simulink model "P702_NI_SoftECU"  (R2019a)
settings: Solver=ode1  StartTime=0.0  StopTime=Inf  FixedStep=0.001  RelTol=1e-3  EnableMultiTasking=on
PreLoadFcn:
  | run '.\VeriStand_BlockSet\NIVeriStandAddPaths.m'
undefined symbols (not defined in the file or in its folder): magnitude
libraries: simulink x83, simulink_extras x1
(part 10 of 76)

== system P702_NI_SoftECU/Input/BCM/Body_Info_4_0x242 ==
  BattULo_I_Actl : S-Function  Priority=1  FunctionName=NIVeriStandIO  Parameters=width dtype portnum stime stype btype  SFunctionDeploymentMode=off  EnableBusSupport=off  mask(NI VeriStand Inport){portnum=1, width=-1, stime=-1, dtype=auto, stype=auto, btype=1}
      mask prompts: portnum "Port number:"; width "Port dimensions (-1 for dynamically sized):"; stime "Sample time (-1 for inherited):"; dtype "Data type:"; stype "Signal type:"; btype "Block type:"
      mask help: Use this inport on any level of nested subsystems to allow NI VeriStand software to map signals to it.
      mask init:
      | NIVeriStandIO_init;
      settings: CopyFcn=NIVeriStand_MDL_functions('', 'IO_copy');  DeleteFcn=NIVeriStand_MDL_functions('', 'IO_delete');  MoveFcn=set_param(gcb, 'Mask', 'on');
      mask Callback portnum: NIVeriStand_MDL_functions('', 'IO_setportnum');
      mask TypeOptions dtype: auto | double | single | int8 | uint8 | int16 | uint16 | int32 | uint32 | boolean
      mask Callback dtype: NIVeriStand_MDL_functions('', 'IO_booleansignal');
      mask TypeOptions stype: auto | real | complex
      mask Display:
      | patch([-x x], [-y y], [.90980 .81960 .32156]);
      | plot([xrad -x x xrad], [yrad -y y yrad]);
      | fprintf('NI In%d', portnum);
  BattULo_U_Actl : S-Function  Priority=2  FunctionName=NIVeriStandIO  Parameters=width dtype portnum stime stype btype  SFunctionDeploymentMode=off  EnableBusSupport=off  mask(NI VeriStand Inport){portnum=2, width=-1, stime=-1, dtype=auto, stype=auto, btype=1}
      mask prompts: portnum "Port number:"; width "Port dimensions (-1 for dynamically sized):"; stime "Sample time (-1 for inherited):"; dtype "Data type:"; stype "Signal type:"; btype "Block type:"
      mask help: Use this inport on any level of nested subsystems to allow NI VeriStand software to map signals to it.
      mask init:
      | NIVeriStandIO_init;
      settings: CopyFcn=NIVeriStand_MDL_functions('', 'IO_copy');  DeleteFcn=NIVeriStand_MDL_functions('', 'IO_delete');  MoveFcn=set_param(gcb, 'Mask', 'on');
      mask Callback portnum: NIVeriStand_MDL_functions('', 'IO_setportnum');
      mask TypeOptions dtype: auto | double | single | int8 | uint8 | int16 | uint16 | int32 | uint32 | boolean
      mask Callback dtype: NIVeriStand_MDL_functions('', 'IO_booleansignal');
      mask TypeOptions stype: auto | real | complex
      mask Display:
      | patch([-x x], [-y y], [.90980 .81960 .32156]);
      | plot([xrad -x x xrad], [yrad -y y yrad]);
      | fprintf('NI In%d', portnum);
  BrkTrnShifLck_B_Stat : S-Function  Priority=3  FunctionName=NIVeriStandIO  Parameters=width dtype portnum stime stype btype  SFunctionDeploymentMode=off  EnableBusSupport=off  mask(NI VeriStand Inport){portnum=3, width=-1, stime=-1, dtype=auto, stype=auto, btype=1}
      mask prompts: portnum "Port number:"; width "Port dimensions (-1 for dynamically sized):"; stime "Sample time (-1 for inherited):"; dtype "Data type:"; stype "Signal type:"; btype "Block type:"
      mask help: Use this inport on any level of nested subsystems to allow NI VeriStand software to map signals to it.
      mask init:
      | NIVeriStandIO_init;
      settings: CopyFcn=NIVeriStand_MDL_functions('', 'IO_copy');  DeleteFcn=NIVeriStand_MDL_functions('', 'IO_delete');  MoveFcn=set_param(gcb, 'Mask', 'on');
      mask Callback portnum: NIVeriStand_MDL_functions('', 'IO_setportnum');
      mask TypeOptions dtype: auto | double | single | int8 | uint8 | int16 | uint16 | int32 | uint32 | boolean
      mask Callback dtype: NIVeriStand_MDL_functions('', 'IO_booleansignal');
      mask TypeOptions stype: auto | real | complex
      mask Display:
      | patch([-x x], [-y y], [.90980 .81960 .32156]);
      | plot([xrad -x x xrad], [yrad -y y yrad]);
      | fprintf('NI In%d', portnum);
  Bus_Sig : BusCreator  Inputs=15
  DcacElPw_D_Rq : S-Function  Priority=4  FunctionName=NIVeriStandIO  Parameters=width dtype portnum stime stype btype  SFunctionDeploymentMode=off  EnableBusSupport=off  mask(NI VeriStand Inport){portnum=4, width=-1, stime=-1, dtype=auto, stype=auto, btype=1}
      mask prompts: portnum "Port number:"; width "Port dimensions (-1 for dynamically sized):"; stime "Sample time (-1 for inherited):"; dtype "Data type:"; stype "Signal type:"; btype "Block type:"
      mask help: Use this inport on any level of nested subsystems to allow NI VeriStand software to map signals to it.
      mask init:
      | NIVeriStandIO_init;
      settings: CopyFcn=NIVeriStand_MDL_functions('', 'IO_copy');  DeleteFcn=NIVeriStand_MDL_functions('', 'IO_delete');  MoveFcn=set_param(gcb, 'Mask', 'on');
      mask Callback portnum: NIVeriStand_MDL_functions('', 'IO_setportnum');
      mask TypeOptions dtype: auto | double | single | int8 | uint8 | int16 | uint16 | int32 | uint32 | boolean
      mask Callback dtype: NIVeriStand_MDL_functions('', 'IO_booleansignal');
      mask TypeOptions stype: auto | real | complex
      mask Display:
      | patch([-x x], [-y y], [.90980 .81960 .32156]);
      | plot([xrad -x x xrad], [yrad -y y yrad]);
      | fprintf('NI In%d', portnum);
  DriverCrankingReq : S-Function  Priority=5  FunctionName=NIVeriStandIO  Parameters=width dtype portnum stime stype btype  SFunctionDeploymentMode=off  EnableBusSupport=off  mask(NI VeriStand Inport){portnum=5, width=-1, stime=-1, dtype=auto, stype=auto, btype=1}
      mask prompts: portnum "Port number:"; width "Port dimensions (-1 for dynamically sized):"; stime "Sample time (-1 for inherited):"; dtype "Data type:"; stype "Signal type:"; btype "Block type:"
      mask help: Use this inport on any level of nested subsystems to allow NI VeriStand software to map signals to it.
      mask init:
      | NIVeriStandIO_init;
      settings: CopyFcn=NIVeriStand_MDL_functions('', 'IO_copy');  DeleteFcn=NIVeriStand_MDL_functions('', 'IO_delete');  MoveFcn=set_param(gcb, 'Mask', 'on');
      mask Callback portnum: NIVeriStand_MDL_functions('', 'IO_setportnum');
      mask TypeOptions dtype: auto | double | single | int8 | uint8 | int16 | uint16 | int32 | uint32 | boolean
      mask Callback dtype: NIVeriStand_MDL_functions('', 'IO_booleansignal');
      mask TypeOptions stype: auto | real | complex
      mask Display:
      | patch([-x x], [-y y], [.90980 .81960 .32156]);
      | plot([xrad -x x xrad], [yrad -y y yrad]);
      | fprintf('NI In%d', portnum);
  EngOff_T_Actl : S-Function  Priority=6  FunctionName=NIVeriStandIO  Parameters=width dtype portnum stime stype btype  SFunctionDeploymentMode=off  EnableBusSupport=off  mask(NI VeriStand Inport){portnum=6, width=-1, stime=-1, dtype=auto, stype=auto, btype=1}
      mask prompts: portnum "Port number:"; width "Port dimensions (-1 for dynamically sized):"; stime "Sample time (-1 for inherited):"; dtype "Data type:"; stype "Signal type:"; btype "Block type:"
      mask help: Use this inport on any level of nested subsystems to allow NI VeriStand software to map signals to it.
      mask init:
      | NIVeriStandIO_init;
      settings: CopyFcn=NIVeriStand_MDL_functions('', 'IO_copy');  DeleteFcn=NIVeriStand_MDL_functions('', 'IO_delete');  MoveFcn=set_param(gcb, 'Mask', 'on');
      mask Callback portnum: NIVeriStand_MDL_functions('', 'IO_setportnum');
      mask TypeOptions dtype: auto | double | single | int8 | uint8 | int16 | uint16 | int32 | uint32 | boolean
      mask Callback dtype: NIVeriStand_MDL_functions('', 'IO_booleansignal');
      mask TypeOptions stype: auto | real | complex
      mask Display:
      | patch([-x x], [-y y], [.90980 .81960 .32156]);
      | plot([xrad -x x xrad], [yrad -y y yrad]);
      | fprintf('NI In%d', portnum);
  FuelPumpPwr_D_Stat : S-Function  Priority=7  FunctionName=NIVeriStandIO  Parameters=width dtype portnum stime stype btype  SFunctionDeploymentMode=off  EnableBusSupport=off  mask(NI VeriStand Inport){portnum=7, width=-1, stime=-1, dtype=auto, stype=auto, btype=1}
      mask prompts: portnum "Port number:"; width "Port dimensions (-1 for dynamically sized):"; stime "Sample time (-1 for inherited):"; dtype "Data type:"; stype "Signal type:"; btype "Block type:"
      mask help: Use this inport on any level of nested subsystems to allow NI VeriStand software to map signals to it.
      mask init:
      | NIVeriStandIO_init;
      settings: CopyFcn=NIVeriStand_MDL_functions('', 'IO_copy');  DeleteFcn=NIVeriStand_MDL_functions('', 'IO_delete');  MoveFcn=set_param(gcb, 'Mask', 'on');
      mask Callback portnum: NIVeriStand_MDL_functions('', 'IO_setportnum');
      mask TypeOptions dtype: auto | double | single | int8 | uint8 | int16 | uint16 | int32 | uint32 | boolean
      mask Callback dtype: NIVeriStand_MDL_functions('', 'IO_booleansignal');
      mask TypeOptions stype: auto | real | complex
      mask Display:
      | patch([-x x], [-y y], [.90980 .81960 .32156]);
      | plot([xrad -x x xrad], [yrad -y y yrad]);
      | fprintf('NI In%d', portnum);
  PrkLckCtlAvail_T_Stat : S-Function  Priority=8  FunctionName=NIVeriStandIO  Parameters=width dtype portnum stime stype btype  SFunctionDeploymentMode=off  EnableBusSupport=off  mask(NI VeriStand Inport){portnum=8, width=-1, stime=-1, dtype=auto, stype=auto, btype=1}
      mask prompts: portnum "Port number:"; width "Port dimensions (-1 for dynamically sized):"; stime "Sample time (-1 for inherited):"; dtype "Data type:"; stype "Signal type:"; btype "Block type:"
      mask help: Use this inport on any level of nested subsystems to allow NI VeriStand software to map signals to it.
      mask init:
      | NIVeriStandIO_init;
      settings: CopyFcn=NIVeriStand_MDL_functions('', 'IO_copy');  DeleteFcn=NIVeriStand_MDL_functions('', 'IO_delete');  MoveFcn=set_param(gcb, 'Mask', 'on');
      mask Callback portnum: NIVeriStand_MDL_functions('', 'IO_setportnum');
      mask TypeOptions dtype: auto | double | single | int8 | uint8 | int16 | uint16 | int32 | uint32 | boolean
      mask Callback dtype: NIVeriStand_MDL_functions('', 'IO_booleansignal');
      mask TypeOptions stype: auto | real | complex
      mask Display:
      | patch([-x x], [-y y], [.90980 .81960 .32156]);
      | plot([xrad -x x xrad], [yrad -y y yrad]);
      | fprintf('NI In%d', portnum);
  PrkLckCtlMsgTxt_D_Rq : S-Function  Priority=9  FunctionName=NIVeriStandIO  Parameters=width dtype portnum stime stype btype  SFunctionDeploymentMode=off  EnableBusSupport=off  mask(NI VeriStand Inport){portnum=9, width=-1, stime=-1, dtype=auto, stype=auto, btype=1}
      mask prompts: portnum "Port number:"; width "Port dimensions (-1 for dynamically sized):"; stime "Sample time (-1 for inherited):"; dtype "Data type:"; stype "Signal type:"; btype "Block type:"
      mask help: Use this inport on any level of nested subsystems to allow NI VeriStand software to map signals to it.
      mask init:
      | NIVeriStandIO_init;
      settings: CopyFcn=NIVeriStand_MDL_functions('', 'IO_copy');  DeleteFcn=NIVeriStand_MDL_functions('', 'IO_delete');  MoveFcn=set_param(gcb, 'Mask', 'on');
      mask Callback portnum: NIVeriStand_MDL_functions('', 'IO_setportnum');
      mask TypeOptions dtype: auto | double | single | int8 | uint8 | int16 | uint16 | int32 | uint32 | boolean
      mask Callback dtype: NIVeriStand_MDL_functions('', 'IO_booleansignal');
      mask TypeOptions stype: auto | real | complex
      mask Display:
      | patch([-x x], [-y y], [.90980 .81960 .32156]);
      | plot([xrad -x x xrad], [yrad -y y yrad]);
      | fprintf('NI In%d', portnum);
  PrkLckCtlTow_B_Enbl : S-Function  Priority=10  FunctionName=NIVeriStandIO  Parameters=width dtype portnum stime stype btype  SFunctionDeploymentMode=off  EnableBusSupport=off  mask(NI VeriStand Inport){portnum=10, width=-1, stime=-1, dtype=auto, stype=auto, btype=1}
      mask prompts: portnum "Port number:"; width "Port dimensions (-1 for dynamically sized):"; stime "Sample time (-1 for inherited):"; dtype "Data type:"; stype "Signal type:"; btype "Block type:"
      mask help: Use this inport on any level of nested subsystems to allow NI VeriStand software to map signals to it.
      mask init:
      | NIVeriStandIO_init;
      settings: CopyFcn=NIVeriStand_MDL_functions('', 'IO_copy');  DeleteFcn=NIVeriStand_MDL_functions('', 'IO_delete');  MoveFcn=set_param(gcb, 'Mask', 'on');
      mask Callback portnum: NIVeriStand_MDL_functions('', 'IO_setportnum');
      mask TypeOptions dtype: auto | double | single | int8 | uint8 | int16 | uint16 | int32 | uint32 | boolean
      mask Callback dtype: NIVeriStand_MDL_functions('', 'IO_booleansignal');
      mask TypeOptions stype: auto | real | complex
      mask Display:
      | patch([-x x], [-y y], [.90980 .81960 .32156]);
      | plot([xrad -x x xrad], [yrad -y y yrad]);
      | fprintf('NI In%d', portnum);
  PrkLckCtlUnlck_D_Stat : S-Function  Priority=11  FunctionName=NIVeriStandIO  Parameters=width dtype portnum stime stype btype  SFunctionDeploymentMode=off  EnableBusSupport=off  mask(NI VeriStand Inport){portnum=11, width=-1, stime=-1, dtype=auto, stype=auto, btype=1}
      mask prompts: portnum "Port number:"; width "Port dimensions (-1 for dynamically sized):"; stime "Sample time (-1 for inherited):"; dtype "Data type:"; stype "Signal type:"; btype "Block type:"
      mask help: Use this inport on any level of nested subsystems to allow NI VeriStand software to map signals to it.
      mask init:
      | NIVeriStandIO_init;
      settings: CopyFcn=NIVeriStand_MDL_functions('', 'IO_copy');  DeleteFcn=NIVeriStand_MDL_functions('', 'IO_delete');  MoveFcn=set_param(gcb, 'Mask', 'on');
      mask Callback portnum: NIVeriStand_MDL_functions('', 'IO_setportnum');
      mask TypeOptions dtype: auto | double | single | int8 | uint8 | int16 | uint16 | int32 | uint32 | boolean
      mask Callback dtype: NIVeriStand_MDL_functions('', 'IO_booleansignal');
      mask TypeOptions stype: auto | real | complex
      mask Display:
      | patch([-x x], [-y y], [.90980 .81960 .32156]);
      | plot([xrad -x x xrad], [yrad -y y yrad]);
      | fprintf('NI In%d', portnum);
  PrkLckCtl_B_Enbl : S-Function  Priority=12  FunctionName=NIVeriStandIO  Parameters=width dtype portnum stime stype btype  SFunctionDeploymentMode=off  EnableBusSupport=off  mask(NI VeriStand Inport){portnum=12, width=-1, stime=-1, dtype=auto, stype=auto, btype=1}
      mask prompts: portnum "Port number:"; width "Port dimensions (-1 for dynamically sized):"; stime "Sample time (-1 for inherited):"; dtype "Data type:"; stype "Signal type:"; btype "Block type:"
      mask help: Use this inport on any level of nested subsystems to allow NI VeriStand software to map signals to it.
      mask init:
      | NIVeriStandIO_init;
      settings: CopyFcn=NIVeriStand_MDL_functions('', 'IO_copy');  DeleteFcn=NIVeriStand_MDL_functions('', 'IO_delete');  MoveFcn=set_param(gcb, 'Mask', 'on');
      mask Callback portnum: NIVeriStand_MDL_functions('', 'IO_setportnum');
      mask TypeOptions dtype: auto | double | single | int8 | uint8 | int16 | uint16 | int32 | uint32 | boolean
      mask Callback dtype: NIVeriStand_MDL_functions('', 'IO_booleansignal');
      mask TypeOptions stype: auto | real | complex
      mask Display:
      | patch([-x x], [-y y], [.90980 .81960 .32156]);
      | plot([xrad -x x xrad], [yrad -y y yrad]);
      | fprintf('NI In%d', portnum);
  PtLatchActv_B_RqBcm : S-Function  Priority=13  FunctionName=NIVeriStandIO  Parameters=width dtype portnum stime stype btype  SFunctionDeploymentMode=off  EnableBusSupport=off  mask(NI VeriStand Inport){portnum=13, width=-1, stime=-1, dtype=auto, stype=auto, btype=1}
      mask prompts: portnum "Port number:"; width "Port dimensions (-1 for dynamically sized):"; stime "Sample time (-1 for inherited):"; dtype "Data type:"; stype "Signal type:"; btype "Block type:"
      mask help: Use this inport on any level of nested subsystems to allow NI VeriStand software to map signals to it.
      mask init:
      | NIVeriStandIO_init;
      settings: CopyFcn=NIVeriStand_MDL_functions('', 'IO_copy');  DeleteFcn=NIVeriStand_MDL_functions('', 'IO_delete');  MoveFcn=set_param(gcb, 'Mask', 'on');
      mask Callback portnum: NIVeriStand_MDL_functions('', 'IO_setportnum');
      mask TypeOptions dtype: auto | double | single | int8 | uint8 | int16 | uint16 | int32 | uint32 | boolean
      mask Callback dtype: NIVeriStand_MDL_functions('', 'IO_booleansignal');
      mask TypeOptions stype: auto | real | complex
      mask Display:
      | patch([-x x], [-y y], [.90980 .81960 .32156]);
      | plot([xrad -x x xrad], [yrad -y y yrad]);
      | fprintf('NI In%d', portnum);
  ReFuelSwtchStat_D_Actl : S-Function  Priority=14  FunctionName=NIVeriStandIO  Parameters=width dtype portnum stime stype btype  SFunctionDeploymentMode=off  EnableBusSupport=off  mask(NI VeriStand Inport){portnum=14, width=-1, stime=-1, dtype=auto, stype=auto, btype=1}
      mask prompts: portnum "Port number:"; width "Port dimensions (-1 for dynamically sized):"; stime "Sample time (-1 for inherited):"; dtype "Data type:"; stype "Signal type:"; btype "Block type:"
      mask help: Use this inport on any level of nested subsystems to allow NI VeriStand software to map signals to it.
      mask init:
      | NIVeriStandIO_init;
      settings: CopyFcn=NIVeriStand_MDL_functions('', 'IO_copy');  DeleteFcn=NIVeriStand_MDL_functions('', 'IO_delete');  MoveFcn=set_param(gcb, 'Mask', 'on');
      mask Callback portnum: NIVeriStand_MDL_functions('', 'IO_setportnum');
      mask TypeOptions dtype: auto | double | single | int8 | uint8 | int16 | uint16 | int32 | uint32 | boolean
      mask Callback dtype: NIVeriStand_MDL_functions('', 'IO_booleansignal');
      mask TypeOptions stype: auto | real | complex
      mask Display:
      | patch([-x x], [-y y], [.90980 .81960 .32156]);
      | plot([xrad -x x xrad], [yrad -y y yrad]);
      | fprintf('NI In%d', portnum);
  immoSecureIdleMode : S-Function  Priority=15  FunctionName=NIVeriStandIO  Parameters=width dtype portnum stime stype btype  SFunctionDeploymentMode=off  EnableBusSupport=off  mask(NI VeriStand Inport){portnum=15, width=-1, stime=-1, dtype=auto, stype=auto, btype=1}
      mask prompts: portnum "Port number:"; width "Port dimensions (-1 for dynamically sized):"; stime "Sample time (-1 for inherited):"; dtype "Data type:"; stype "Signal type:"; btype "Block type:"
      mask help: Use this inport on any level of nested subsystems to allow NI VeriStand software to map signals to it.
      mask init:
      | NIVeriStandIO_init;
      settings: CopyFcn=NIVeriStand_MDL_functions('', 'IO_copy');  DeleteFcn=NIVeriStand_MDL_functions('', 'IO_delete');  MoveFcn=set_param(gcb, 'Mask', 'on');
      mask Callback portnum: NIVeriStand_MDL_functions('', 'IO_setportnum');
      mask TypeOptions dtype: auto | double | single | int8 | uint8 | int16 | uint16 | int32 | uint32 | boolean
      mask Callback dtype: NIVeriStand_MDL_functions('', 'IO_booleansignal');
      mask TypeOptions stype: auto | real | complex
      mask Display:
      | patch([-x x], [-y y], [.90980 .81960 .32156]);
      | plot([xrad -x x xrad], [yrad -y y yrad]);
      | fprintf('NI In%d', portnum);
  Body_Info_4_0x242 : Outport
  wires:
  Bus_Sig/1 -> Body_Info_4_0x242/1  "Body_Info_4_0x242"
  BattULo_I_Actl/1 -> Bus_Sig/1  "BattULo_I_Actl"
  BattULo_U_Actl/1 -> Bus_Sig/2  "BattULo_U_Actl"
  BrkTrnShifLck_B_Stat/1 -> Bus_Sig/3  "BrkTrnShifLck_B_Stat"
  DcacElPw_D_Rq/1 -> Bus_Sig/4  "DcacElPw_D_Rq"
  DriverCrankingReq/1 -> Bus_Sig/5  "DriverCrankingReq"
  EngOff_T_Actl/1 -> Bus_Sig/6  "EngOff_T_Actl"
  FuelPumpPwr_D_Stat/1 -> Bus_Sig/7  "FuelPumpPwr_D_Stat"
  PrkLckCtlAvail_T_Stat/1 -> Bus_Sig/8  "PrkLckCtlAvail_T_Stat"
  PrkLckCtlMsgTxt_D_Rq/1 -> Bus_Sig/9  "PrkLckCtlMsgTxt_D_Rq"
  PrkLckCtlTow_B_Enbl/1 -> Bus_Sig/10  "PrkLckCtlTow_B_Enbl"
  PrkLckCtlUnlck_D_Stat/1 -> Bus_Sig/11  "PrkLckCtlUnlck_D_Stat"
  PrkLckCtl_B_Enbl/1 -> Bus_Sig/12  "PrkLckCtl_B_Enbl"
  PtLatchActv_B_RqBcm/1 -> Bus_Sig/13  "PtLatchActv_B_RqBcm"
  ReFuelSwtchStat_D_Actl/1 -> Bus_Sig/14  "ReFuelSwtchStat_D_Actl"
  immoSecureIdleMode/1 -> Bus_Sig/15  "immoSecureIdleMode"

== system P702_NI_SoftECU/Input/BCM/Body_Info_6_0x38D ==
  Bus_Sig : BusCreator  Inputs=15
  DrLatchMsgTxt_D_Rq : Constant  Commented=on  Value=0
  ElPwPoint_D_Rq : Constant  Commented=on  Value=0
  HeadLghtHiPrmsn_D_Stat : Constant  Commented=on  Value=3
  IgnPsswrdDsply_B_Rq : Constant  Commented=on  Value=0
  KeyAdmnTot_No_Cnt : Constant  Commented=on  Value=0
  KeyMykeyTot_No_Cnt : Constant  Commented=on  Value=0
  Keycode_Status : Constant  Commented=on  Value=0
  PEBackupSlot_Stats : Constant  Commented=on  Value=0
  PoliceIdlMde_D_Stat : Constant  Commented=on  Value=0
  PrmtrAlrmEvnt_D_Stat : Constant  Commented=on  Value=0
  PrsnlDevcChrgEnbl_B_Rq : Constant  Commented=on  Value=0
  SecurityMsgTxt_D_Rq : Constant  Commented=on  Value=0
  SteWhlLckMsgTxt_D_Rq : Constant  Commented=on  Value=0
  TracKeyMde_D_Stat : Constant  Commented=on  Value=0
  immoMsgTxt_D_Rq : Constant  Commented=on  Value=0
  Body_Info_6_0x38D : Outport
  wires:
  Bus_Sig/1 -> Body_Info_6_0x38D/1  "Body_Info_6_0x38D"
  KeyAdmnTot_No_Cnt/1 -> Bus_Sig/1  "KeyAdmnTot_No_Cnt"
  KeyMykeyTot_No_Cnt/1 -> Bus_Sig/2  "KeyMykeyTot_No_Cnt"
  Keycode_Status/1 -> Bus_Sig/3  "Keycode_Status"
  PEBackupSlot_Stats/1 -> Bus_Sig/4  "PEBackupSlot_Stats"
  SteWhlLckMsgTxt_D_Rq/1 -> Bus_Sig/5  "SteWhlLckMsgTxt_D_Rq"
  immoMsgTxt_D_Rq/1 -> Bus_Sig/6  "immoMsgTxt_D_Rq"
  PrmtrAlrmEvnt_D_Stat/1 -> Bus_Sig/7  "PrmtrAlrmEvnt_D_Stat"
  SecurityMsgTxt_D_Rq/1 -> Bus_Sig/8  "SecurityMsgTxt_D_Rq"
  TracKeyMde_D_Stat/1 -> Bus_Sig/9  "TracKeyMde_D_Stat"
  DrLatchMsgTxt_D_Rq/1 -> Bus_Sig/10  "DrLatchMsgTxt_D_Rq"
  PrsnlDevcChrgEnbl_B_Rq/1 -> Bus_Sig/11  "PrsnlDevcChrgEnbl_B_Rq"
  PoliceIdlMde_D_Stat/1 -> Bus_Sig/12  "PoliceIdlMde_D_Stat"
  HeadLghtHiPrmsn_D_Stat/1 -> Bus_Sig/13  "HeadLghtHiPrmsn_D_Stat"
  ElPwPoint_D_Rq/1 -> Bus_Sig/14  "ElPwPoint_D_Rq"
  IgnPsswrdDsply_B_Rq/1 -> Bus_Sig/15  "IgnPsswrdDsply_B_Rq"

== system P702_NI_SoftECU/Input/BCM/Body_Info_7_0x3B1 ==
  Bus_Sig : BusCreator  Inputs=1
  KeyOffMde_D_Actl : Constant  Commented=on  Value=0
  Body_Info_7_0x3B1 : Outport
  wires:
  Bus_Sig/1 -> Body_Info_7_0x3B1/1  "Body_Info_7_0x3B1"
  KeyOffMde_D_Actl/1 -> Bus_Sig/1  "KeyOffMde_D_Actl"

== system P702_NI_SoftECU/Input/BCM/Body_Info_8_0x3B9 ==
  Bus_Sig : BusCreator  Inputs=7
  ChrgCordLck_B_Stat : Constant  Commented=on  Value=0
  ChrgCordResp1_No_Actl : Constant  Commented=on  Value=0
  ChrgCordResp2_No_Actl : Constant  Commented=on  Value=0
  WakeAlarm0_D_Stat : Constant  Commented=on  Value=3
  WakeAlarm1_D_Stat : Constant  Commented=on  Value=3
  WakeAlarm2_D_Stat : Constant  Commented=on  Value=3
  WakeAlarm3_D_Stat : Constant  Commented=on  Value=3
  Body_Info_8_0x3B9 : Outport
  wires:
  Bus_Sig/1 -> Body_Info_8_0x3B9/1  "Body_Info_8_0x3B9"
  WakeAlarm0_D_Stat/1 -> Bus_Sig/1  "WakeAlarm0_D_Stat"
  WakeAlarm1_D_Stat/1 -> Bus_Sig/2  "WakeAlarm1_D_Stat"
  WakeAlarm2_D_Stat/1 -> Bus_Sig/3  "WakeAlarm2_D_Stat"
  WakeAlarm3_D_Stat/1 -> Bus_Sig/4  "WakeAlarm3_D_Stat"
  ChrgCordResp1_No_Actl/1 -> Bus_Sig/5  "ChrgCordResp1_No_Actl"
  ChrgCordResp2_No_Actl/1 -> Bus_Sig/6  "ChrgCordResp2_No_Actl"
  ChrgCordLck_B_Stat/1 -> Bus_Sig/7  "ChrgCordLck_B_Stat"

== system P702_NI_SoftECU/Input/BCM/Body_Info_9_0x3A3 ==
  AdvStrt_D_Stat : Constant  Commented=on  Value=0
  Bus_Sig : BusCreator  Inputs=10
  CrnkInhbt_B_Stat : Constant  Commented=on
  CrnkInhbt_No_Cnt : Constant  Commented=on  Value=0
  CrnkInhbt_No_Cs : Constant  Commented=on  Value=0
  DrvInCtl_B_Stat : Constant  Commented=on  Value=0
  EngStrtActv_B_Stat : Constant  Commented=on  Value=0
  EngStrt_B_Rq : Constant  Commented=on  Value=0
  IgnPreOffActv_B_Stat : Constant  Commented=on  Value=0
  StrtrMtrCtlDStat_No_Cs : Constant  Commented=on  Value=0
  VehOnSrc_D_Stat : Constant  Commented=on  Value=0
  Body_Info_9_0x3A3 : Outport
  wires:
  Bus_Sig/1 -> Body_Info_9_0x3A3/1  "Body_Info_9_0x3A3"
  CrnkInhbt_B_Stat/1 -> Bus_Sig/1  "CrnkInhbt_B_Stat"
  CrnkInhbt_No_Cnt/1 -> Bus_Sig/2  "CrnkInhbt_No_Cnt"
  IgnPreOffActv_B_Stat/1 -> Bus_Sig/3  "IgnPreOffActv_B_Stat"
  DrvInCtl_B_Stat/1 -> Bus_Sig/4  "DrvInCtl_B_Stat"
  EngStrt_B_Rq/1 -> Bus_Sig/5  "EngStrt_B_Rq"
  CrnkInhbt_No_Cs/1 -> Bus_Sig/6  "CrnkInhbt_No_Cs"
  AdvStrt_D_Stat/1 -> Bus_Sig/7  "AdvStrt_D_Stat"
  VehOnSrc_D_Stat/1 -> Bus_Sig/8  "VehOnSrc_D_Stat"
  StrtrMtrCtlDStat_No_Cs/1 -> Bus_Sig/9  "StrtrMtrCtlDStat_No_Cs"
  EngStrtActv_B_Stat/1 -> Bus_Sig/10  "EngStrtActv_B_Stat"

== system P702_NI_SoftECU/Input/BCM/CMPS_FDM_Info_Status_0x3C7 ==
  Bus_Sig : BusCreator  Inputs=7
  CamPDCGuidStat : Constant  Commented=on  Value=0
  CamZoomActiveState : Constant  Commented=on  Value=0
  CamraOvrlDyn_D_Actl : Constant  Commented=on  Value=0
  CamraOvrlStat_D_Actl : Constant  Commented=on  Value=0
  CamraOvrlTow_D_Actl : Constant  Commented=on  Value=0
  CamraViewSplit_D_Actl : Constant  Commented=on  Value=2
  CamraZoomMan_D_Actl : Constant  Commented=on  Value=0
  CMPS_FDM_Info_Status_0x3C7 : Outport
  wires:
  Bus_Sig/1 -> CMPS_FDM_Info_Status_0x3C7/1  "CMPS_FDM_Info_Status_0x3C7"
  CamraViewSplit_D_Actl/1 -> Bus_Sig/1  "CamraViewSplit_D_Actl"
  CamraOvrlDyn_D_Actl/1 -> Bus_Sig/2  "CamraOvrlDyn_D_Actl"
  CamraZoomMan_D_Actl/1 -> Bus_Sig/3  "CamraZoomMan_D_Actl"
  CamPDCGuidStat/1 -> Bus_Sig/4  "CamPDCGuidStat"
  CamZoomActiveState/1 -> Bus_Sig/5  "CamZoomActiveState"
  CamraOvrlStat_D_Actl/1 -> Bus_Sig/6  "CamraOvrlStat_D_Actl"
  CamraOvrlTow_D_Actl/1 -> Bus_Sig/7  "CamraOvrlTow_D_Actl"

== system P702_NI_SoftECU/Input/BCM/CellPhonePassport_Stat_1_0x447 ==
  Bus_Sig : BusCreator  Inputs=11
  HeadLghtOn_D_Rq : Constant  Commented=on
  KeyProg_No_Actl : Constant  Commented=on  Value=0
  PepsKeyActv_D_Stat : Constant  Commented=on  Value=0
  PepsKeyFound_No_Actl : Constant  Commented=on  Value=0
  Pers1Phone_D_Stat : Constant  Commented=on  Value=0
  Pers2Phone_D_Stat : Constant  Commented=on  Value=0
  Pers3Phone_D_Stat : Constant  Commented=on  Value=0
  Pers4Phone_D_Stat : Constant  Commented=on  Value=0
  RstrtSetting_T_Actl : Constant  Commented=on  Value=0
  Rstrt_T_Actl : Constant  Commented=on  Value=0
  VehLck_D_Dsply : Constant  Commented=on  Value=0
  CellPhonePassport_Stat_1_0x447 : Outport
  wires:
  Bus_Sig/1 -> CellPhonePassport_Stat_1_0x447/1  "CellPhonePassport_Stat_1_0x447"
  KeyProg_No_Actl/1 -> Bus_Sig/1  "KeyProg_No_Actl"
  PepsKeyActv_D_Stat/1 -> Bus_Sig/2  "PepsKeyActv_D_Stat"
  Rstrt_T_Actl/1 -> Bus_Sig/3  "Rstrt_T_Actl"
  RstrtSetting_T_Actl/1 -> Bus_Sig/4  "RstrtSetting_T_Actl"
  PepsKeyFound_No_Actl/1 -> Bus_Sig/5  "PepsKeyFound_No_Actl"
  HeadLghtOn_D_Rq/1 -> Bus_Sig/6  "HeadLghtOn_D_Rq"
  VehLck_D_Dsply/1 -> Bus_Sig/7  "VehLck_D_Dsply"
  Pers1Phone_D_Stat/1 -> Bus_Sig/8  "Pers1Phone_D_Stat"
  Pers2Phone_D_Stat/1 -> Bus_Sig/9  "Pers2Phone_D_Stat"
  Pers3Phone_D_Stat/1 -> Bus_Sig/10  "Pers3Phone_D_Stat"
  Pers4Phone_D_Stat/1 -> Bus_Sig/11  "Pers4Phone_D_Stat"

== system P702_NI_SoftECU/Input/BCM/GGCC_Config_Mgmt_ID_1_0x40A ==
  Bus_Sig : BusCreator  Inputs=1
  VehicleGGCCData : Constant  Commented=on  Value=0
  GGCC_Config_Mgmt_ID_1_0x40A : Outport
  wires:
  Bus_Sig/1 -> GGCC_Config_Mgmt_ID_1_0x40A/1  "GGCC_Config_Mgmt_ID_1_0x40A"
  VehicleGGCCData/1 -> Bus_Sig/1  "VehicleGGCCData"

== system P702_NI_SoftECU/Input/BCM/GlobalClock_Data_0x84 ==
  Bus_Sig : BusCreator  Inputs=5
  GlblClkDay_No_Actl_In : S-Function  Priority=1  FunctionName=NIVeriStandIO  Parameters=width dtype portnum stime stype btype  SFunctionDeploymentMode=off  EnableBusSupport=off  mask(NI VeriStand Inport){portnum=1, width=-1, stime=-1, dtype=auto, stype=auto, btype=1}
      mask prompts: portnum "Port number:"; width "Port dimensions (-1 for dynamically sized):"; stime "Sample time (-1 for inherited):"; dtype "Data type:"; stype "Signal type:"; btype "Block type:"
      mask help: Use this inport on any level of nested subsystems to allow NI VeriStand software to map signals to it.
      mask init:
      | NIVeriStandIO_init;
      settings: CopyFcn=NIVeriStand_MDL_functions('', 'IO_copy');  DeleteFcn=NIVeriStand_MDL_functions('', 'IO_delete');  MoveFcn=set_param(gcb, 'Mask', 'on');
      mask Callback portnum: NIVeriStand_MDL_functions('', 'IO_setportnum');
      mask TypeOptions dtype: auto | double | single | int8 | uint8 | int16 | uint16 | int32 | uint32 | boolean
      mask Callback dtype: NIVeriStand_MDL_functions('', 'IO_booleansignal');
      mask TypeOptions stype: auto | real | complex
      mask Display:
      | patch([-x x], [-y y], [.90980 .81960 .32156]);
      | plot([xrad -x x xrad], [yrad -y y yrad]);
      | fprintf('NI In%d', portnum);
  GlblClkHr_No_Actl_In : S-Function  Priority=2  FunctionName=NIVeriStandIO  Parameters=width dtype portnum stime stype btype  SFunctionDeploymentMode=off  EnableBusSupport=off  mask(NI VeriStand Inport){portnum=2, width=-1, stime=-1, dtype=auto, stype=auto, btype=1}
      mask prompts: portnum "Port number:"; width "Port dimensions (-1 for dynamically sized):"; stime "Sample time (-1 for inherited):"; dtype "Data type:"; stype "Signal type:"; btype "Block type:"
      mask help: Use this inport on any level of nested subsystems to allow NI VeriStand software to map signals to it.
      mask init:
      | NIVeriStandIO_init;
      settings: CopyFcn=NIVeriStand_MDL_functions('', 'IO_copy');  DeleteFcn=NIVeriStand_MDL_functions('', 'IO_delete');  MoveFcn=set_param(gcb, 'Mask', 'on');
      mask Callback portnum: NIVeriStand_MDL_functions('', 'IO_setportnum');
      mask TypeOptions dtype: auto | double | single | int8 | uint8 | int16 | uint16 | int32 | uint32 | boolean
      mask Callback dtype: NIVeriStand_MDL_functions('', 'IO_booleansignal');
      mask TypeOptions stype: auto | real | complex
      mask Display:
      | patch([-x x], [-y y], [.90980 .81960 .32156]);
      | plot([xrad -x x xrad], [yrad -y y yrad]);
      | fprintf('NI In%d', portnum);
  GlblClkMnte_No_Actl_In : S-Function  Priority=3  FunctionName=NIVeriStandIO  Parameters=width dtype portnum stime stype btype  SFunctionDeploymentMode=off  EnableBusSupport=off  mask(NI VeriStand Inport){portnum=3, width=-1, stime=-1, dtype=auto, stype=auto, btype=1}
      mask prompts: portnum "Port number:"; width "Port dimensions (-1 for dynamically sized):"; stime "Sample time (-1 for inherited):"; dtype "Data type:"; stype "Signal type:"; btype "Block type:"
      mask help: Use this inport on any level of nested subsystems to allow NI VeriStand software to map signals to it.
      mask init:
      | NIVeriStandIO_init;
      settings: CopyFcn=NIVeriStand_MDL_functions('', 'IO_copy');  DeleteFcn=NIVeriStand_MDL_functions('', 'IO_delete');  MoveFcn=set_param(gcb, 'Mask', 'on');
      mask Callback portnum: NIVeriStand_MDL_functions('', 'IO_setportnum');
      mask TypeOptions dtype: auto | double | single | int8 | uint8 | int16 | uint16 | int32 | uint32 | boolean
      mask Callback dtype: NIVeriStand_MDL_functions('', 'IO_booleansignal');
      mask TypeOptions stype: auto | real | complex
      mask Display:
      | patch([-x x], [-y y], [.90980 .81960 .32156]);
      | plot([xrad -x x xrad], [yrad -y y yrad]);
      | fprintf('NI In%d', portnum);
  GlblClkScnd_No_Actl_In : S-Function  Priority=4  FunctionName=NIVeriStandIO  Parameters=width dtype portnum stime stype btype  SFunctionDeploymentMode=off  EnableBusSupport=off  mask(NI VeriStand Inport){portnum=4, width=-1, stime=-1, dtype=auto, stype=auto, btype=1}
      mask prompts: portnum "Port number:"; width "Port dimensions (-1 for dynamically sized):"; stime "Sample time (-1 for inherited):"; dtype "Data type:"; stype "Signal type:"; btype "Block type:"
      mask help: Use this inport on any level of nested subsystems to allow NI VeriStand software to map signals to it.
      mask init:
      | NIVeriStandIO_init;
      settings: CopyFcn=NIVeriStand_MDL_functions('', 'IO_copy');  DeleteFcn=NIVeriStand_MDL_functions('', 'IO_delete');  MoveFcn=set_param(gcb, 'Mask', 'on');
      mask Callback portnum: NIVeriStand_MDL_functions('', 'IO_setportnum');
      mask TypeOptions dtype: auto | double | single | int8 | uint8 | int16 | uint16 | int32 | uint32 | boolean
      mask Callback dtype: NIVeriStand_MDL_functions('', 'IO_booleansignal');
      mask TypeOptions stype: auto | real | complex
      mask Display:
      | patch([-x x], [-y y], [.90980 .81960 .32156]);
      | plot([xrad -x x xrad], [yrad -y y yrad]);
      | fprintf('NI In%d', portnum);
  GlblClkYr_No_Actl_In : S-Function  Priority=5  FunctionName=NIVeriStandIO  Parameters=width dtype portnum stime stype btype  SFunctionDeploymentMode=off  EnableBusSupport=off  mask(NI VeriStand Inport){portnum=5, width=-1, stime=-1, dtype=auto, stype=auto, btype=1}
      mask prompts: portnum "Port number:"; width "Port dimensions (-1 for dynamically sized):"; stime "Sample time (-1 for inherited):"; dtype "Data type:"; stype "Signal type:"; btype "Block type:"
      mask help: Use this inport on any level of nested subsystems to allow NI VeriStand software to map signals to it.
      mask init:
      | NIVeriStandIO_init;
      settings: CopyFcn=NIVeriStand_MDL_functions('', 'IO_copy');  DeleteFcn=NIVeriStand_MDL_functions('', 'IO_delete');  MoveFcn=set_param(gcb, 'Mask', 'on');
      mask Callback portnum: NIVeriStand_MDL_functions('', 'IO_setportnum');
      mask TypeOptions dtype: auto | double | single | int8 | uint8 | int16 | uint16 | int32 | uint32 | boolean
      mask Callback dtype: NIVeriStand_MDL_functions('', 'IO_booleansignal');
      mask TypeOptions stype: auto | real | complex
      mask Display:
      | patch([-x x], [-y y], [.90980 .81960 .32156]);
      | plot([xrad -x x xrad], [yrad -y y yrad]);
      | fprintf('NI In%d', portnum);
  GlobalClock_Data_0x84 : Outport
  wires:
  Bus_Sig/1 -> GlobalClock_Data_0x84/1  "GlobalClock_Data_0x84"
  GlblClkYr_No_Actl_In/1 -> Bus_Sig/1  "GlblClkYr_No_Actl"
  GlblClkDay_No_Actl_In/1 -> Bus_Sig/2  "GlblClkDay_No_Actl"
  GlblClkMnte_No_Actl_In/1 -> Bus_Sig/3  "GlblClkMnte_No_Actl"
  GlblClkScnd_No_Actl_In/1 -> Bus_Sig/4  "GlblClkScnd_No_Actl"
  GlblClkHr_No_Actl_In/1 -> Bus_Sig/5  "GlblClkHr_No_Actl"

== system P702_NI_SoftECU/Input/BCM/Global_PATS_Control_Info2_0x42 ==
  Bus_Sig : BusCreator  Inputs=2
  immoControlCmd_T2 : Constant  Commented=on  Value=0
  immoControlData_T2 : Constant  Commented=on  Value=0
  Global_PATS_Control_Info2_0x42 : Outport
  wires:
  Bus_Sig/1 -> Global_PATS_Control_Info2_0x42/1  "Global_PATS_Control_Info2_0x42"
  immoControlCmd_T2/1 -> Bus_Sig/1  "immoControlCmd_T2"
  immoControlData_T2/1 -> Bus_Sig/2  "immoControlData_T2"

== system P702_NI_SoftECU/Input/BCM/Global_PATS_Control_Info_0x41 ==
  Bus_Sig : BusCreator  Inputs=2
  immoControlCmd_T1 : Constant  Commented=on  Value=0
  immoControlData_T1 : Constant  Commented=on  Value=0
  Global_PATS_Control_Info_0x41 : Outport
  wires:
  Bus_Sig/1 -> Global_PATS_Control_Info_0x41/1  "Global_PATS_Control_Info_0x41"
  immoControlCmd_T1/1 -> Bus_Sig/1  "immoControlCmd_T1"
  immoControlData_T1/1 -> Bus_Sig/2  "immoControlData_T1"

== system P702_NI_SoftECU/Input/BCM/Locking_Systems_2_0x331 ==
  Bus_Sig : BusCreator  Inputs=20
  ChildLckMde_B_Stat : Constant  Commented=on  Value=0
  ChildLck_D_Dsply : Constant  Commented=on
  DrTgateExtSwMde_B_Stat : Constant  Commented=on  Value=0
  DrTgateOpen_B_Rq : Constant  Commented=on  Value=0
  FobComm_D_Stat : Constant  Commented=on  Value=0
  Keyfob_Pad_Msg_Count : Constant  Commented=on  Value=0
  L_Pwr_Sliding_Dr_Rqst : Constant  Commented=on  Value=0
  LockInhibit : Constant  Commented=on  Value=0
  Lockmsgtxt_D_Rq : Constant  Commented=on  Value=0
  Power_Decklid_Rqst : Constant  Commented=on  Value=0
  Power_Liftgate_Rqst : Constant  Commented=on  Value=0
  R_Pwr_Sliding_Dr_Rqst : Constant  Commented=on  Value=0
  Remote_Device_Feedback : Constant  Commented=on  Value=0
  RollCodeUnlock : Constant  Commented=on  Value=0
  VehLckInd_D_Rq : Constant  Commented=on  Value=0
  Veh_Lock_EvNum : Constant  Commented=on  Value=0
  Veh_Lock_Requestor : Constant  Commented=on  Value=0
  Veh_Lock_Status : Constant  Commented=on
  Veh_Lock_Sub_Id : Constant  Commented=on  Value=0
  WindowLockout_B_Stat : Constant  Commented=on  Value=0
  Locking_Systems_2_0x331 : Outport
  wires:
  Bus_Sig/1 -> Locking_Systems_2_0x331/1  "Locking_Systems_2_0x331"
  ChildLck_D_Dsply/1 -> Bus_Sig/1  "ChildLck_D_Dsply"
  FobComm_D_Stat/1 -> Bus_Sig/2  "FobComm_D_Stat"
  L_Pwr_Sliding_Dr_Rqst/1 -> Bus_Sig/3  "L_Pwr_Sliding_Dr_Rqst"
  LockInhibit/1 -> Bus_Sig/4  "LockInhibit"
  Power_Decklid_Rqst/1 -> Bus_Sig/5  "Power_Decklid_Rqst"
  Power_Liftgate_Rqst/1 -> Bus_Sig/6  "Power_Liftgate_Rqst"
  Keyfob_Pad_Msg_Count/1 -> Bus_Sig/7  "Keyfob_Pad_Msg_Count"
  RollCodeUnlock/1 -> Bus_Sig/8  "RollCodeUnlock"
  Lockmsgtxt_D_Rq/1 -> Bus_Sig/9  "Lockmsgtxt_D_Rq"
  R_Pwr_Sliding_Dr_Rqst/1 -> Bus_Sig/10  "R_Pwr_Sliding_Dr_Rqst"
  WindowLockout_B_Stat/1 -> Bus_Sig/11  "WindowLockout_B_Stat"
  Veh_Lock_Status/1 -> Bus_Sig/12  "Veh_Lock_Status"
  DrTgateExtSwMde_B_Stat/1 -> Bus_Sig/13  "DrTgateExtSwMde_B_Stat"
  Veh_Lock_EvNum/1 -> Bus_Sig/14  "Veh_Lock_EvNum"
  Veh_Lock_Requestor/1 -> Bus_Sig/15  "Veh_Lock_Requestor"
  Remote_Device_Feedback/1 -> Bus_Sig/16  "Remote_Device_Feedback"
  Veh_Lock_Sub_Id/1 -> Bus_Sig/17  "Veh_Lock_Sub_Id"
  DrTgateOpen_B_Rq/1 -> Bus_Sig/18  "DrTgateOpen_B_Rq"
  VehLckInd_D_Rq/1 -> Bus_Sig/19  "VehLckInd_D_Rq"
  ChildLckMde_B_Stat/1 -> Bus_Sig/20  "ChildLckMde_B_Stat"

== system P702_NI_SoftECU/Input/BCM/PaakRqData1_0x468 ==
  Bus_Sig : BusCreator  Inputs=6
  KeyPadCodeProg_D_Stat : Constant  Commented=on  Value=0
  PaakTrgtData_D_Rq : Constant  Commented=on  Value=0
  PaakTrgtPssvData_No_Rq : Constant  Commented=on  Value=0
  PaakTrgtRollCode_No_Rq : Constant  Commented=on  Value=0
  PaakTrgtType_D_Rq : Constant  Commented=on  Value=0
  PaakTrgtZone_D_Rq : Constant  Commented=on  Value=0
  PaakRqData1_0x468 : Outport
  wires:
  Bus_Sig/1 -> PaakRqData1_0x468/1  "PaakRqData1_0x468"
  PaakTrgtPssvData_No_Rq/1 -> Bus_Sig/1  "PaakTrgtPssvData_No_Rq"
  PaakTrgtData_D_Rq/1 -> Bus_Sig/2  "PaakTrgtData_D_Rq"
  PaakTrgtRollCode_No_Rq/1 -> Bus_Sig/3  "PaakTrgtRollCode_No_Rq"
  PaakTrgtType_D_Rq/1 -> Bus_Sig/4  "PaakTrgtType_D_Rq"
  PaakTrgtZone_D_Rq/1 -> Bus_Sig/5  "PaakTrgtZone_D_Rq"
  KeyPadCodeProg_D_Stat/1 -> Bus_Sig/6  "KeyPadCodeProg_D_Stat"

== system P702_NI_SoftECU/Input/BCM/PaakRqData2_0x469 ==
  Bus_Sig : BusCreator  Inputs=1
  PaakTrgtActvData_No_Rq : Constant  Commented=on  Value=0
  PaakRqData2_0x469 : Outport
  wires:
  Bus_Sig/1 -> PaakRqData2_0x469/1  "PaakRqData2_0x469"
  PaakTrgtActvData_No_Rq/1 -> Bus_Sig/1  "PaakTrgtActvData_No_Rq"

== system P702_NI_SoftECU/Input/BCM/Personality_BCM2_Data_0x3EB ==
  AssocConfirm_D_Actl : Constant  Commented=on  Value=0
  Bus_Sig : BusCreator  Inputs=16
  EmPrflKeyAssoc_D_Stat : Constant  Commented=on  Value=0
  EmPrflNo_D_Stat : Constant  Commented=on  Value=0
  Pers1Key_D_Stat : Constant  Commented=on  Value=0
  Pers2Key_D_Stat : Constant  Commented=on  Value=0
  Pers3Key_D_Stat : Constant  Commented=on  Value=0
  Pers4Key_D_Stat : Constant  Commented=on  Value=0
  PersConflict_D_Actl : Constant  Commented=on
  PersNoPos_D_Actl : Constant  Commented=on  Value=4
  PersNo_D_Actl : Constant  Commented=on  Value=4
  PersRecallSrc_D_Actl : Constant  Commented=on  Value=0
  PersSetupAccessCtrl : Constant  Commented=on  Value=0
  PersSetupRestr_D_Actl : Constant  Commented=on  Value=0
  PersSetup_No_Actl : Constant  Commented=on  Value=0
  RecallEvent_No_Cnt : Constant  Commented=on  Value=0
  VehKeyActv_D_Stat : Constant  Commented=on  Value=0
  Personality_BCM2_Data_0x3EB : Outport
  wires:
  Bus_Sig/1 -> Personality_BCM2_Data_0x3EB/1  "Personality_BCM2_Data_0x3EB"
  RecallEvent_No_Cnt/1 -> Bus_Sig/1  "RecallEvent_No_Cnt"
  AssocConfirm_D_Actl/1 -> Bus_Sig/2  "AssocConfirm_D_Actl"
  Pers1Key_D_Stat/1 -> Bus_Sig/3  "Pers1Key_D_Stat"
  PersNo_D_Actl/1 -> Bus_Sig/4  "PersNo_D_Actl"
  PersConflict_D_Actl/1 -> Bus_Sig/5  "PersConflict_D_Actl"
  PersSetupRestr_D_Actl/1 -> Bus_Sig/6  "PersSetupRestr_D_Actl"
  PersSetupAccessCtrl/1 -> Bus_Sig/7  "PersSetupAccessCtrl"
  PersNoPos_D_Actl/1 -> Bus_Sig/8  "PersNoPos_D_Actl"
  PersSetup_No_Actl/1 -> Bus_Sig/9  "PersSetup_No_Actl"
  VehKeyActv_D_Stat/1 -> Bus_Sig/10  "VehKeyActv_D_Stat"
  Pers2Key_D_Stat/1 -> Bus_Sig/11  "Pers2Key_D_Stat"
  Pers3Key_D_Stat/1 -> Bus_Sig/12  "Pers3Key_D_Stat"
  EmPrflKeyAssoc_D_Stat/1 -> Bus_Sig/13  "EmPrflKeyAssoc_D_Stat"
  EmPrflNo_D_Stat/1 -> Bus_Sig/14  "EmPrflNo_D_Stat"
  Pers4Key_D_Stat/1 -> Bus_Sig/15  "Pers4Key_D_Stat"
  PersRecallSrc_D_Actl/1 -> Bus_Sig/16  "PersRecallSrc_D_Actl"

== system P702_NI_SoftECU/Input/BCM/Personality_BCM_Data_0x3E3 ==
  Bus_Sig : BusCreator  Inputs=6
  FeatConfigBcmActl : Constant  Commented=on  Value=0
  FeatNoBcm_No_Actl : Constant  Commented=on  Value=0
  FobAssocChime_B_Rq : Constant  Commented=on  Value=0
  LightAmbColor_No_Actl : Constant  Commented=on  Value=0
  LightAmbIntsty_No_Actl : Constant  Commented=on  Value=0
  PersIndexBcm_D_Actl : Constant  Commented=on  Value=4
  Personality_BCM_Data_0x3E3 : Outport
  wires:
  Bus_Sig/1 -> Personality_BCM_Data_0x3E3/1  "Personality_BCM_Data_0x3E3"
  FeatConfigBcmActl/1 -> Bus_Sig/1  "FeatConfigBcmActl"
  FeatNoBcm_No_Actl/1 -> Bus_Sig/2  "FeatNoBcm_No_Actl"
  PersIndexBcm_D_Actl/1 -> Bus_Sig/3  "PersIndexBcm_D_Actl"
  FobAssocChime_B_Rq/1 -> Bus_Sig/4  "FobAssocChime_B_Rq"
  LightAmbColor_No_Actl/1 -> Bus_Sig/5  "LightAmbColor_No_Actl"
  LightAmbIntsty_No_Actl/1 -> Bus_Sig/6  "LightAmbIntsty_No_Actl"

== system P702_NI_SoftECU/Input/BCM/Power_Stat_0x456 ==
  Bus_Sig : BusCreator  Inputs=1
  RstrnMdulePw_D_Falt : Constant  Commented=on
  Power_Stat_0x456 : Outport
  wires:
  Bus_Sig/1 -> Power_Stat_0x456/1  "Power_Stat_0x456"
  RstrnMdulePw_D_Falt/1 -> Bus_Sig/1  "RstrnMdulePw_D_Falt"

== system P702_NI_SoftECU/Input/BCM/RKE_Packet_0x3B6 ==
  Bus_Sig : BusCreator  Inputs=6
  Modulation_Ctrl : Constant  Commented=on  Value=0
  RemoteKey_Info_Ctrl : Constant  Commented=on  Value=0
  RemoteKey_Info_Index : Constant  Commented=on  Value=0
  RemoteKey_Info_MaxInd : Constant  Commented=on  Value=0
  RemoteKey_Info_TIC : Constant  Commented=on  Value=0
  TirePress_Filter_Ctrl : Constant  Commented=on  Value=2
  RKE_Packet_0x3B6 : Outport
  wires:
  Bus_Sig/1 -> RKE_Packet_0x3B6/1  "RKE_Packet_0x3B6"
  TirePress_Filter_Ctrl/1 -> Bus_Sig/1  "TirePress_Filter_Ctrl"
  Modulation_Ctrl/1 -> Bus_Sig/2  "Modulation_Ctrl"
  RemoteKey_Info_Ctrl/1 -> Bus_Sig/3  "RemoteKey_Info_Ctrl"
  RemoteKey_Info_Index/1 -> Bus_Sig/4  "RemoteKey_Info_Index"
  RemoteKey_Info_MaxInd/1 -> Bus_Sig/5  "RemoteKey_Info_MaxInd"
  RemoteKey_Info_TIC/1 -> Bus_Sig/6  "RemoteKey_Info_TIC"

== system P702_NI_SoftECU/Input/BCM/TPM_Frame_0x3B7 ==
  Bus_Sig : BusCreator  Inputs=3
  TirePress_Info_ID : Constant  Commented=on  Value=0
  TirePress_Info_Index : Constant  Commented=on  Value=0
  TirePress_Info_MaxInd : Constant  Commented=on  Value=0
  TPM_Frame_0x3B7 : Outport
  wires:
  Bus_Sig/1 -> TPM_Frame_0x3B7/1  "TPM_Frame_0x3B7"
  TirePress_Info_Index/1 -> Bus_Sig/1  "TirePress_Info_Index"
  TirePress_Info_MaxInd/1 -> Bus_Sig/2  "TirePress_Info_MaxInd"
  TirePress_Info_ID/1 -> Bus_Sig/3  "TirePress_Info_ID"

== system P702_NI_SoftECU/Input/BCM/Tire_Pressure_Data_0x3B5 ==
  Bus_Sig : BusCreator  Inputs=4
  Tire_Press_LF_Data : Constant  Commented=on  Value=65533
  Tire_Press_LR_OLR_Data : Constant  Commented=on  Value=65533
  Tire_Press_RF_Data : Constant  Commented=on  Value=65533
  Tire_Press_RR_ORR_Data : Constant  Commented=on  Value=65533
  Tire_Pressure_Data_0x3B5 : Outport
  wires:
  Bus_Sig/1 -> Tire_Pressure_Data_0x3B5/1  "Tire_Pressure_Data_0x3B5"
  Tire_Press_LF_Data/1 -> Bus_Sig/1  "Tire_Press_LF_Data"
  Tire_Press_RF_Data/1 -> Bus_Sig/2  "Tire_Press_RF_Data"
  Tire_Press_RR_ORR_Data/1 -> Bus_Sig/3  "Tire_Press_RR_ORR_Data"
  Tire_Press_LR_OLR_Data/1 -> Bus_Sig/4  "Tire_Press_LR_OLR_Data"

== system P702_NI_SoftECU/Input/BCM/Tire_Pressure_Data_DRW_0x3B8 ==
  Bus_Sig : BusCreator  Inputs=2
  Tire_Press_ILR_Data : Constant  Commented=on  Value=65533
  Tire_Press_IRR_Data : Constant  Commented=on  Value=65533
  Tire_Pressure_Data_DRW_0x3B8 : Outport
  wires:
  Bus_Sig/1 -> Tire_Pressure_Data_DRW_0x3B8/1  "Tire_Pressure_Data_DRW_0x3B8"
  Tire_Press_ILR_Data/1 -> Bus_Sig/1  "Tire_Press_ILR_Data"
  Tire_Press_IRR_Data/1 -> Bus_Sig/2  "Tire_Press_IRR_Data"

== system P702_NI_SoftECU/Input/BCM/Tire_Pressure_Stat_0x3B4 ==
  Bus_Sig : BusCreator  Inputs=11
  TirePReset_D_Stat : Constant  Commented=on  Value=0
  Tire_Press_ILR_Stat : Constant  Commented=on  Value=0
  Tire_Press_IRR_Stat : Constant  Commented=on  Value=0
  Tire_Press_LF_Stat : Constant  Commented=on  Value=0
  Tire_Press_LR_OLR_Stat : Constant  Commented=on  Value=0
  Tire_Press_Placrd_Frnt : Constant  Commented=on  Value=255
  Tire_Press_Placrd_Rear : Constant  Commented=on  Value=255
  Tire_Press_RF_Stat : Constant  Commented=on  Value=0
  Tire_Press_RR_ORR_Stat : Constant  Commented=on  Value=0
  Tire_Press_System_Stat : Constant  Commented=on  Value=0
  Tire_Press_Telltale : Constant  Commented=on  Value=0
  Tire_Pressure_Stat_0x3B4 : Outport
  wires:
  Bus_Sig/1 -> Tire_Pressure_Stat_0x3B4/1  "Tire_Pressure_Stat_0x3B4"
  Tire_Press_System_Stat/1 -> Bus_Sig/1  "Tire_Press_System_Stat"
  Tire_Press_Telltale/1 -> Bus_Sig/2  "Tire_Press_Telltale"
  TirePReset_D_Stat/1 -> Bus_Sig/3  "TirePReset_D_Stat"
  Tire_Press_LF_Stat/1 -> Bus_Sig/4  "Tire_Press_LF_Stat"
  Tire_Press_RF_Stat/1 -> Bus_Sig/5  "Tire_Press_RF_Stat"
  Tire_Press_RR_ORR_Stat/1 -> Bus_Sig/6  "Tire_Press_RR_ORR_Stat"
  Tire_Press_LR_OLR_Stat/1 -> Bus_Sig/7  "Tire_Press_LR_OLR_Stat"
  Tire_Press_IRR_Stat/1 -> Bus_Sig/8  "Tire_Press_IRR_Stat"
  Tire_Press_ILR_Stat/1 -> Bus_Sig/9  "Tire_Press_ILR_Stat"
  Tire_Press_Placrd_Frnt/1 -> Bus_Sig/10  "Tire_Press_Placrd_Frnt"
  Tire_Press_Placrd_Rear/1 -> Bus_Sig/11  "Tire_Press_Placrd_Rear"
